simulink model "state_feedback"  (R2015b)
settings: Solver=VariableStepAuto  StartTime=0.0  StopTime=5000*0.02  RelTol=1e-3
values from neighbouring files (symbols this model uses):
  A12 = A(1:3,4:6)    [StateSpace.m]
  F = Fe(:,1:size(A,2))    [StateSpace.m]
  FI = Fe(:,size(A,2)+1:size(Fe,2))    [StateSpace.m]
  Lobs = (-place(A22',A12',[-11 -12 -13]))'    [StateSpace.m]
undefined symbols (not defined in the file or in its folder): Jx, Jy, Jz, kd, kth, L, w1_bar, w2_bar, w3_bar, w4_bar
settings Model: Creator=USUARIO  LastModifiedBy=USUARIO

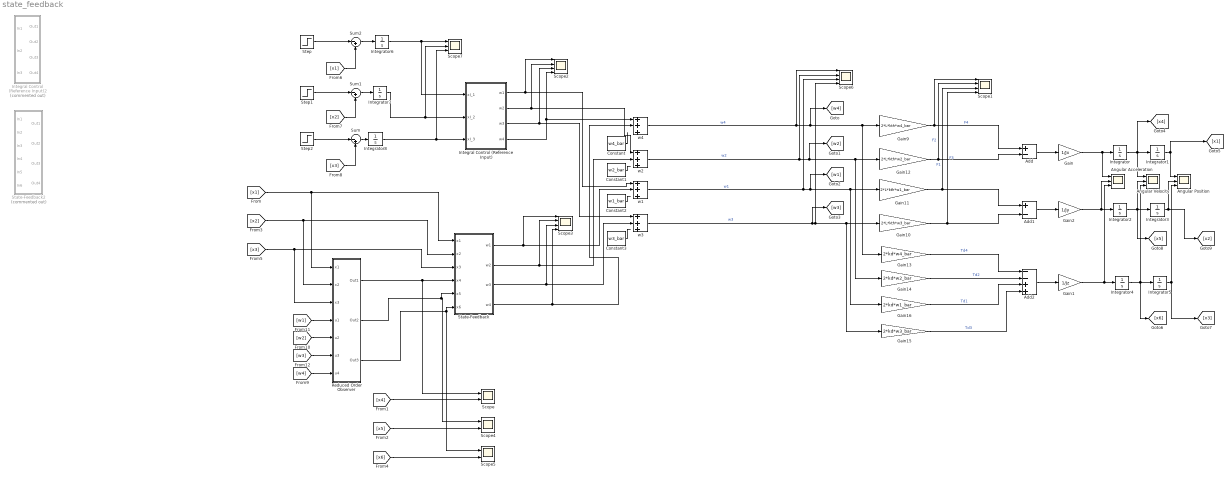
== system state_feedback ==
  Add : Sum  Inputs=+-
  Add1 : Sum  Inputs=+-
  Add2 : Sum  Inputs=--++
  Angular Position : Scope  NumInputPorts=3
  Angular Velocity : Scope  NumInputPorts=3
  Angular Acceleration : Scope  NumInputPorts=3
  Constant : Constant  Value=w4_bar
  Constant1 : Constant  Value=w2_bar
  Constant2 : Constant  Value=w1_bar
  Constant3 : Constant  Value=w3_bar
  Gain : Gain  Gain=1/Jx
  Gain1 : Gain  Gain=1/Jz
  Gain10 : Gain  Gain=2*L*kth*w3_bar
  Gain11 : Gain  Gain=2*L*kth*w1_bar
  Gain12 : Gain  Gain=2*L*kth*w2_bar
  Gain13 : Gain  Gain=2*kd*w4_bar
  Gain14 : Gain  Gain=2*kd*w2_bar
  Gain15 : Gain  Gain=2*kd*w3_bar
  Gain16 : Gain  Gain=2*kd*w1_bar
  Gain2 : Gain  Gain=1/Jy
  Gain9 : Gain  Gain=2*L*kth*w4_bar
  Integral Control (Reference Input) : MATLAB Function  TreatAsAtomicUnit=on
  Integral Control (Reference Input)2 : Subsystem  Commented=on
  Integrator{,1..8} (9 alike) : Integrator
  Reduced Order Observer : Subsystem
  Scope : Scope  NumInputPorts=2
  Scope{1..3,6} (4 alike) : Scope  NumInputPorts=4
  Scope4 : Scope  NumInputPorts=2
  Scope5 : Scope  NumInputPorts=2
  Scope7 : Scope  NumInputPorts=3
  "State-Feedback " : MATLAB Function  TreatAsAtomicUnit=on
  State-Feedback2 : Subsystem  Commented=on
  Step : Step  Time=5  After=0.5  SampleTime=0
  Step1 : Step  Time=5  After=0  SampleTime=0
  Step2 : Step  Time=5  After=0  SampleTime=0
  Sum : Sum  Inputs=|-+
  Sum1 : Sum  Inputs=|-+
  Sum2 : Sum  Inputs=|-+
  w{1..4} (4 alike) : Sum  Inputs=+++
  wires:
  Add2/1 -> Gain1/1
  Add1/1 -> Gain2/1
  Add/1 -> Gain/1
  Gain/1 -> Angular Acceleration/1, Integrator/1
  Gain2/1 -> Angular Acceleration/2, Integrator2/1
  Gain1/1 -> Integrator4/1, Angular Acceleration/3
  Integrator4/1 -> Angular Velocity/3, [x6], Integrator5/1
  Integrator2/1 -> Angular Velocity/2, [x5], Integrator3/1
  Integrator/1 -> [x4], Angular Velocity/1, Integrator1/1
  Integrator3/1 -> [x2], Angular Position/2
  Gain9/1 -> Add/1, Scope1/1  "F4"
  Gain12/1 -> Scope1/2, Add/2  "F2"
  Gain10/1 -> Scope1/4, Add1/2  "F3"
  Gain11/1 -> Scope1/3, Add1/1  "F1"
  Gain14/1 -> Add2/2  "Td2"
  Gain13/1 -> Add2/1  "Td4"
  Gain16/1 -> Add2/3  "Td1"
  Gain15/1 -> Add2/4  "Td3"
  w4/1 -> Scope6/1, Gain9/1, Gain13/1, [w4]  "w4"
  Step2/1 -> Sum/1
  Step1/1 -> Sum1/1
  [x1] -> Sum2/2
  [x2] -> Sum1/2
  [x3] -> Sum/2
  Sum2/1 -> Integrator6/1
  Sum1/1 -> Integrator7/1
  Sum/1 -> Integrator8/1
  "State-Feedback "/1(w1) -> w1/2, Scope3/1
  "State-Feedback "/2(w2) -> w2/2, Scope3/2
  "State-Feedback "/4(w4) -> w4/2, Scope3/4
  Integral Control (Reference Input)/1(w1) -> w1/1, Scope2/1
  Integral Control (Reference Input)/2(w2) -> w2/1, Scope2/2
  Integral Control (Reference Input)/3(w3) -> w3/1, Scope2/3
  Integral Control (Reference Input)/4(w4) -> Scope2/4, w4/1
  "State-Feedback "/3(w3) -> w3/2, Scope3/3
  [w1] -> Reduced Order Observer/4(u1)
  [w2] -> Reduced Order Observer/5(u2)
  [w3] -> Reduced Order Observer/6(u3)
  [w4] -> Reduced Order Observer/7(u4)
  Reduced Order Observer/1(Out1) -> "State-Feedback "/4(x4), Scope/1
  Reduced Order Observer/2(Out2) -> "State-Feedback "/5(x5), Scope4/1
  Reduced Order Observer/3(Out3) -> "State-Feedback "/6(x6), Scope5/1
  [x4] -> Scope/2
  [x5] -> Scope4/2
  [x6] -> Scope5/2
  w2/1 -> Scope6/2, Gain12/1, Gain14/1, [w2]  "w2"
  w3/1 -> Scope6/4, Gain15/1, Gain10/1, [w3]  "w3"
  w1/1 -> Scope6/3, Gain11/1, Gain16/1, [w1]  "w1"
  Constant/1 -> ?
  Constant1/1 -> ?
  Constant2/1 -> ?
  Constant3/1 -> ?
  Step/1 -> Sum2/1
  Integrator1/1 -> Angular Position/1, [x1]
  Integrator5/1 -> Angular Position/3, [x3]
  Integrator6/1 -> Integral Control (Reference Input)/1(xI_1), Scope7/1
  Integrator7/1 -> Scope7/2, Integral Control (Reference Input)/2(xI_2)
  Integrator8/1 -> Scope7/3, Integral Control (Reference Input)/3(xI_3)
  [x1] -> "State-Feedback "/1(x1), Reduced Order Observer/1(x1)
  [x2] -> "State-Feedback "/2(x2), Reduced Order Observer/2(x2)
  [x3] -> "State-Feedback "/3(x3), Reduced Order Observer/3(x3)

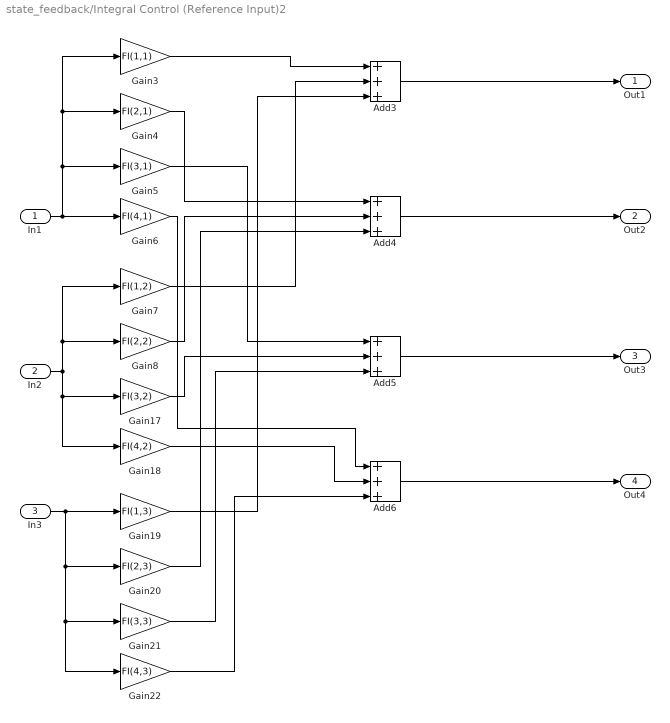
== system state_feedback/Integral Control (Reference Input)2 ==
  In1 : Inport
  In2 : Inport  Port=2
  In3 : Inport  Port=3
  Add{3..6} (4 alike) : Sum  Inputs=+++
  Gain17 : Gain  Gain=FI(3,2)
  Gain18 : Gain  Gain=FI(4,2)
  Gain19 : Gain  Gain=FI(1,3)
  Gain20 : Gain  Gain=FI(2,3)
  Gain21 : Gain  Gain=FI(3,3)
  Gain22 : Gain  Gain=FI(4,3)
  Gain3 : Gain  Gain=FI(1,1)
  Gain4 : Gain  Gain=FI(2,1)
  Gain5 : Gain  Gain=FI(3,1)
  Gain6 : Gain  Gain=FI(4,1)
  Gain7 : Gain  Gain=FI(1,2)
  Gain8 : Gain  Gain=FI(2,2)
  Out1 : Outport
  Out2 : Outport  Port=2
  Out3 : Outport  Port=3
  Out4 : Outport  Port=4
  wires:
  Gain21/1 -> Add5/3
  Gain17/1 -> Add5/2
  Gain5/1 -> Add5/1
  Gain6/1 -> Add6/1
  Gain22/1 -> Add6/3
  Gain18/1 -> Add6/2
  In2/1 -> Gain7/1, Gain8/1, Gain17/1, Gain18/1
  Add5/1 -> Out3/1
  Add6/1 -> Out4/1
  In3/1 -> Gain19/1, Gain20/1, Gain22/1, Gain21/1
  Add3/1 -> Out1/1
  Add4/1 -> Out2/1
  Gain20/1 -> Add4/3
  Gain3/1 -> Add3/1
  Gain19/1 -> Add3/3
  Gain7/1 -> Add3/2
  Gain8/1 -> Add4/2
  Gain4/1 -> Add4/1
  In1/1 -> Gain3/1, Gain4/1, Gain5/1, Gain6/1

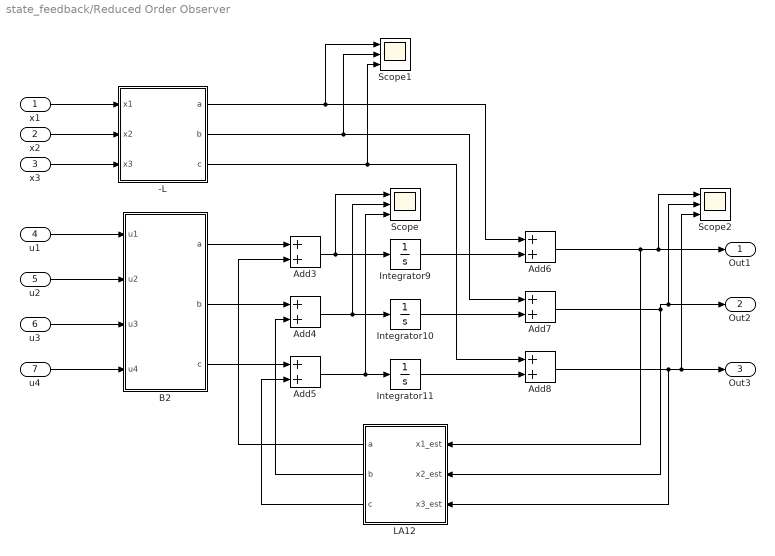
== system state_feedback/Reduced Order Observer ==
  x1 : Inport
  x2 : Inport  Port=2
  x3 : Inport  Port=3
  u1 : Inport  Port=4
  u2 : Inport  Port=5
  u3 : Inport  Port=6
  u4 : Inport  Port=7
  "-L " : MATLAB Function  TreatAsAtomicUnit=on
  Add{3..8} (6 alike) : Sum  Inputs=2
  B2 : MATLAB Function  TreatAsAtomicUnit=on
  Integrator10 : Integrator
  Integrator11 : Integrator
  Integrator9 : Integrator
  LA12 : MATLAB Function  TreatAsAtomicUnit=on
  Scope : Scope  NumInputPorts=3
  Scope1 : Scope  NumInputPorts=3
  Scope2 : Scope  NumInputPorts=3
  Out1 : Outport
  Out2 : Outport  Port=2
  Out3 : Outport  Port=3
  wires:
  u4/1 -> B2/4(u4)
  u2/1 -> B2/2(u2)
  B2/1(a) -> Add3/1
  B2/2(b) -> Add4/1
  B2/3(c) -> Add5/1
  LA12/1(a) -> Add3/2
  LA12/2(b) -> Add4/2
  LA12/3(c) -> Add5/2
  "-L "/3(c) -> Scope1/3, Add8/1
  "-L "/1(a) -> Scope1/1, Add6/1
  "-L "/2(b) -> Scope1/2, Add7/1
  x2/1 -> "-L "/2(x2)
  x3/1 -> "-L "/3(x3)
  x1/1 -> "-L "/1(x1)
  u1/1 -> B2/1(u1)
  u3/1 -> B2/3(u3)
  Add5/1 -> Integrator11/1, Scope/3
  Add3/1 -> Integrator9/1, Scope/1
  Add4/1 -> Integrator10/1, Scope/2
  Integrator9/1 -> Add6/2
  Integrator10/1 -> Add7/2
  Integrator11/1 -> Add8/2
  Add6/1 -> LA12/1(x1_est), Scope2/1, Out1/1
  Add7/1 -> LA12/2(x2_est), Scope2/2, Out2/1
  Add8/1 -> LA12/3(x3_est), Scope2/3, Out3/1

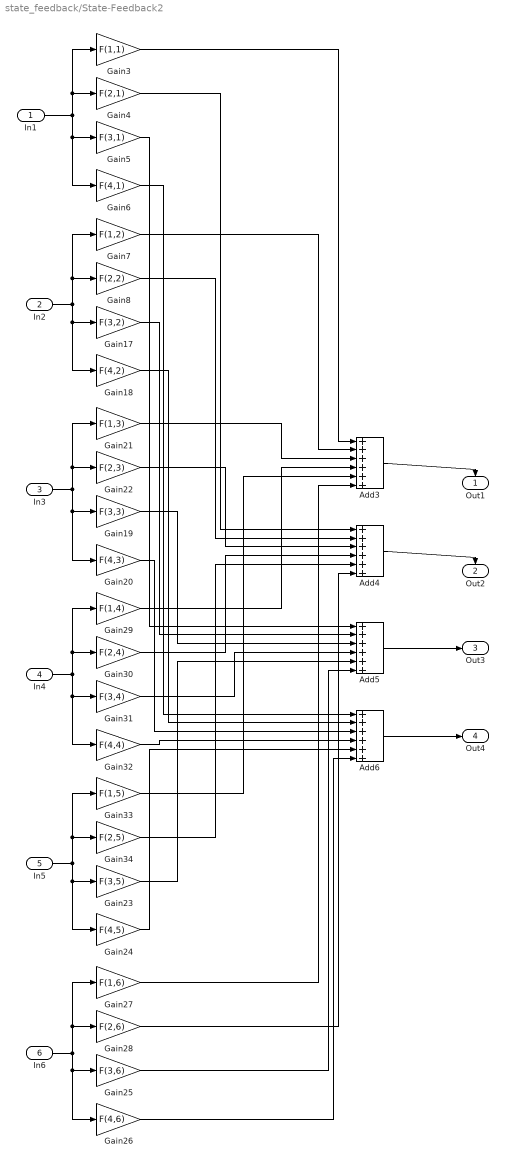
== system state_feedback/State-Feedback2 ==
  In1 : Inport
  In2 : Inport  Port=2
  In3 : Inport  Port=3
  In4 : Inport  Port=4
  In5 : Inport  Port=5
  In6 : Inport  Port=6
  Add{3..6} (4 alike) : Sum  Inputs=++++++
  Gain17 : Gain  Gain=F(3,2)
  Gain18 : Gain  Gain=F(4,2)
  Gain19 : Gain  Gain=F(3,3)
  Gain20 : Gain  Gain=F(4,3)
  Gain21 : Gain  Gain=F(1,3)
  Gain22 : Gain  Gain=F(2,3)
  Gain23 : Gain  Gain=F(3,5)
  Gain24 : Gain  Gain=F(4,5)
  Gain25 : Gain  Gain=F(3,6)
  Gain26 : Gain  Gain=F(4,6)
  Gain27 : Gain  Gain=F(1,6)
  Gain28 : Gain  Gain=F(2,6)
  Gain29 : Gain  Gain=F(1,4)
  Gain3 : Gain  Gain=F(1,1)
  Gain30 : Gain  Gain=F(2,4)
  Gain31 : Gain  Gain=F(3,4)
  Gain32 : Gain  Gain=F(4,4)
  Gain33 : Gain  Gain=F(1,5)
  Gain34 : Gain  Gain=F(2,5)
  Gain4 : Gain  Gain=F(2,1)
  Gain5 : Gain  Gain=F(3,1)
  Gain6 : Gain  Gain=F(4,1)
  Gain7 : Gain  Gain=F(1,2)
  Gain8 : Gain  Gain=F(2,2)
  Out1 : Outport
  Out2 : Outport  Port=2
  Out3 : Outport  Port=3
  Out4 : Outport  Port=4
  wires:
  In2/1 -> Gain8/1, Gain7/1, Gain18/1, Gain17/1
  In1/1 -> Gain6/1, Gain5/1, Gain4/1, Gain3/1
  In3/1 -> Gain22/1, Gain21/1, Gain20/1, Gain19/1
  In5/1 -> Gain34/1, Gain33/1, Gain24/1, Gain23/1
  In4/1 -> Gain32/1, Gain31/1, Gain30/1, Gain29/1
  In6/1 -> Gain28/1, Gain27/1, Gain26/1, Gain25/1
  Add3/1 -> Out1/1
  Add4/1 -> Out2/1
  Add5/1 -> Out3/1
  Add6/1 -> Out4/1
  Gain4/1 -> Add4/1
  Gain22/1 -> Add4/3
  Gain8/1 -> Add4/2
  Gain34/1 -> Add4/5
  Gain30/1 -> Add4/4
  Gain28/1 -> Add4/6
  Gain24/1 -> Add6/5
  Gain20/1 -> Add6/3
  Gain6/1 -> Add6/1
  Gain18/1 -> Add6/2
  Gain26/1 -> Add6/6
  Gain32/1 -> Add6/4
  Gain7/1 -> Add3/2
  Gain21/1 -> Add3/3
  Gain29/1 -> Add3/4
  Gain27/1 -> Add3/6
  Gain3/1 -> Add3/1
  Gain33/1 -> Add3/5
  Gain23/1 -> Add5/5
  Gain17/1 -> Add5/2
  Gain19/1 -> Add5/3
  Gain5/1 -> Add5/1
  Gain31/1 -> Add5/4
  Gain25/1 -> Add5/6

== matlab function state_feedback/State-Feedback  ==
  data: x1 input; w1 output; w2 output; w3 output; w4 output; x2 input; x3 input; x4 input; x5 input; x6 input; F parameter
function [w1,w2,w3,w4] = F_matrix(x1, x2, x3, x4, x5, x6, F)
x=[x1;
    x2;
    x3;
    x4;
    x5;
    x6];

w=F*x;

w1=w(1);
w2=w(2);
w3=w(3);
w4=w(4);

== matlab function state_feedback/Integral Control (Reference Input) ==
  data: xI_1 input; w1 output; w2 output; w3 output; w4 output; xI_2 input; xI_3 input; FI parameter
function [w1,w2,w3,w4] = FI_matrix(xI_1, xI_2, xI_3,FI)
xI=[xI_1;
    xI_2;
    xI_3];

w=FI*xI;

w1=w(1);
w2=w(2);
w3=w(3);
w4=w(4);

== matlab function state_feedback/Reduced Order Observer/-L  ==
  data: x1 input; a output; b output; c output; x2 input; x3 input; Lobs parameter
function [a,b,c] = minusL_matrix(x1, x2, x3, Lobs)
x=[x1;
    x2;
    x3];

abc=-Lobs*x;

a=abc(1);
b=abc(2);
c=abc(3);

== matlab function state_feedback/Reduced Order Observer/B2 ==
  data: u1 input; a output; b output; c output; u2 input; u3 input; u4 input; B2 parameter
function [a, b, c] = B2_matrix(u1, u2, u3, u4, B2)
u=[u1;
    u2;
    u3;
    u4];

abc=B2*u;

a=abc(1);
b=abc(2);
c=abc(3);

== matlab function state_feedback/Reduced Order Observer/LA12 ==
  data: x1_est input; x2_est input; x3_est input; a output; b output; c output; Lobs parameter; A12 parameter
function [a,b,c] = LA12_matrix(x1_est, x2_est, x3_est, Lobs, A12)
x=[x1_est;
    x2_est;
    x3_est];

abc=Lobs*A12*x;

a=abc(1);
b=abc(2);
c=abc(3);
